simulink model "fluidDynamicSurface_th"  (R2018b)
settings: Solver=VariableStepAuto  StartTime=0.0  StopTime=0  RelTol=1e-3
undefined symbols (not defined in the file): angVelBdy, ctrlSurfDefl, velCMBdy, velWindBdy
libraries: fluidDynamicSurface_cl x1
settings Model: Creator=mcobb  LastModifiedBy=mcobb

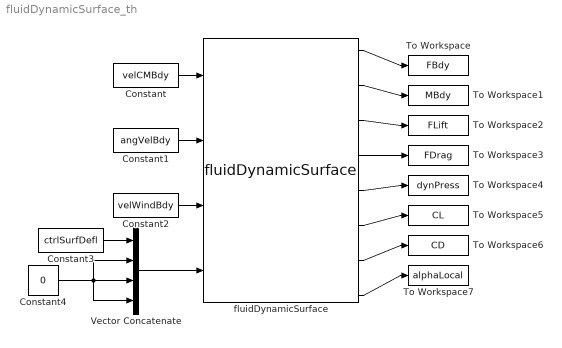
== system fluidDynamicSurface_th ==
  Constant : Constant  Value=velCMBdy
  Constant1 : Constant  Value=angVelBdy
  Constant2 : Constant  Value=velWindBdy
  Constant3 : Constant  Value=ctrlSurfDefl
  Constant4 : Constant  Value=0
  To Workspace : ToWorkspace  VariableName=FBdy  SaveFormat=Timeseries  SampleTime=-1
  To Workspace1 : ToWorkspace  VariableName=MBdy  SaveFormat=Timeseries  SampleTime=-1
  To Workspace2 : ToWorkspace  VariableName=FLift  SaveFormat=Timeseries  SampleTime=-1
  To Workspace3 : ToWorkspace  VariableName=FDrag  SaveFormat=Timeseries  SampleTime=-1
  To Workspace4 : ToWorkspace  VariableName=dynPress  SaveFormat=Timeseries  SampleTime=-1
  To Workspace5 : ToWorkspace  VariableName=CL  SaveFormat=Timeseries  SampleTime=-1
  To Workspace6 : ToWorkspace  VariableName=CD  SaveFormat=Timeseries  SampleTime=-1
  To Workspace7 : ToWorkspace  VariableName=alphaLocal  SaveFormat=Timeseries  SampleTime=-1
  Vector Concatenate : Concatenate  NumInputs=4
  fluidDynamicSurface : fluidDynamicSurface_cl/fluidDynamicSurface  aeroStruct=aeroStruct  fluidDensity=1000
  wires:
  fluidDynamicSurface/1 -> To Workspace/1
  Constant/1 -> fluidDynamicSurface/1
  Constant1/1 -> fluidDynamicSurface/2
  Constant2/1 -> fluidDynamicSurface/3
  Constant3/1 -> Vector Concatenate/1
  fluidDynamicSurface/3 -> To Workspace2/1
  fluidDynamicSurface/4 -> To Workspace3/1
  Vector Concatenate/1 -> fluidDynamicSurface/4
  Constant4/1 -> Vector Concatenate/4, Vector Concatenate/3, Vector Concatenate/2
  fluidDynamicSurface/2 -> To Workspace1/1
  fluidDynamicSurface/5 -> To Workspace4/1
  fluidDynamicSurface/6 -> To Workspace5/1
  fluidDynamicSurface/7 -> To Workspace6/1
  fluidDynamicSurface/8 -> To Workspace7/1
